simulink model "fs9_sim_sdr_v1"  (R2022b)
settings: Solver=ode4  StartTime=0.0  StopTime=dm.duration  FixedStep=dm.dt  RelTol=1e-3
PreLoadFcn:
  | addpath('./Common');
  | addpath('./design_tuning');
  | addpath('./sim_config');
  | addpath('./sim_analysis');
  | addpath('./fsw_init');
  | addpath('./mdls');
  | rads2rpm    = 60/(2*pi);  %rad/s to rpm
  | deg2rad     = pi/180;
  | set_mdl_variant;
InitFcn:
  | %b5g_init_param_sdr_v1;
model workspace (MAT data in the model file):
  RWModelType = 0
undefined symbols (not defined in the file or in its folder): dm, Eclipse, fsw, MagSc, mdl, PVeci, Qi2b, RateSc, SunSc
libraries: simulink x3, vrlib x2, aerolibtransform2 x1
(part 1 of 2)
Description:
  | This is a simplified model for B5G AOCS design and verification.
settings Model: SimulationMode=accelerator  PacingRate=501  ParameterArgumentNames=RWModelType  Creator=Jack-AOCS  LastModifiedBy=toby
settings SolverCC: AlgebraicLoopSolver=TrustRegion  MinimalZcImpactIntegration=on
settings DataIOCC: SaveFormat=Array
settings OptimizationCC: AccelVerboseBuild=on
settings DebuggingCC: ReadBeforeWriteMsg=DisableAll  WriteAfterWriteMsg=DisableAll  WriteAfterReadMsg=DisableAll  MultiTaskDSMMsg=none  UnconnectedInputMsg=warning  UnconnectedOutputMsg=warning  UnconnectedLineMsg=warning  SFMachineParentedDataDiag=warning  ArithmeticOperatorsInVariantConditions=warning
settings ModelReferenceCC: UpdateModelReferenceTargets=IfOutOfDate  EnableRefExpFcnMdlSchedulingChecks=on
settings SFSimCC: SFSimEcho=off  SimUseLocalCustomCode=off  CustomCodeUndefinedFunction=UseInterfaceOnly
settings RTWCC: RTWUseLocalCustomCode=off  DLArmComputeVersion=19.05

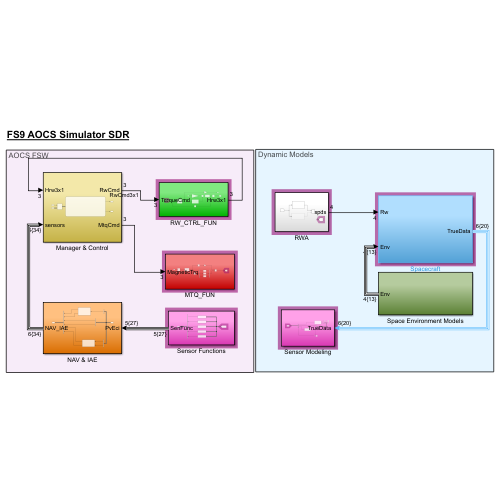
[thumbnail: Simulink's stored preview of the top-level diagram]
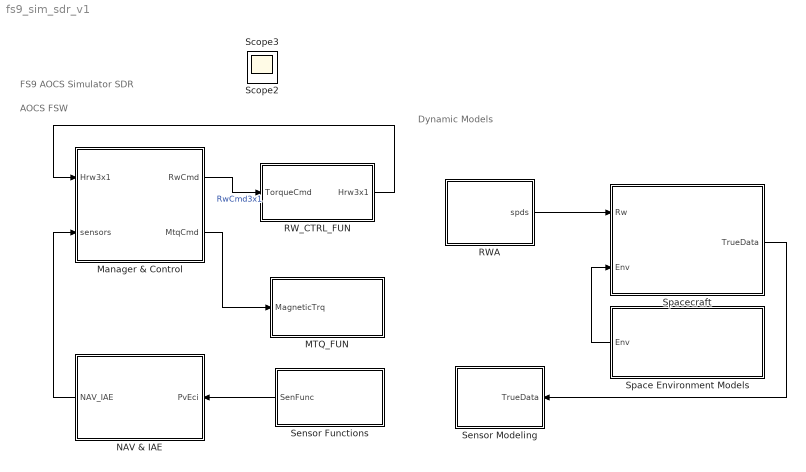
== system fs9_sim_sdr_v1 ==
  note: FS9 AOCS Simulator SDR
  note: AOCS FSW
  note: Dynamic Models
  MTQ_FUN : Subsystem
  Manager & Control : Subsystem
  NAV & IAE : Subsystem
  RWA : Subsystem
  RW_CTRL_FUN : Subsystem
  Sensor Functions : Subsystem
  Sensor Modeling : Subsystem
  Space Environment Models : Subsystem
  Spacecraft : Subsystem
  Scope2 : Scope
  Scope3 : Scope
  wires:
  RWA/1(spds) -> Spacecraft/1(Rw)
  Space Environment Models/1(Env) -> Spacecraft/2(Env)
  Spacecraft/1(TrueData) -> Sensor Modeling/1("TrueData ")
  RW_CTRL_FUN/1(Hrw3x1) -> Manager & Control/1(Hrw3x1)
  NAV & IAE/1(NAV_IAE) -> Manager & Control/2(sensors)
  Manager & Control/1(RwCmd) -> RW_CTRL_FUN/1(TorqueCmd)  "RwCmd3x1"
  Manager & Control/2(MtqCmd) -> MTQ_FUN/1(MagneticTrq)
  Sensor Functions/1(SenFunc) -> NAV & IAE/1(PvEci)

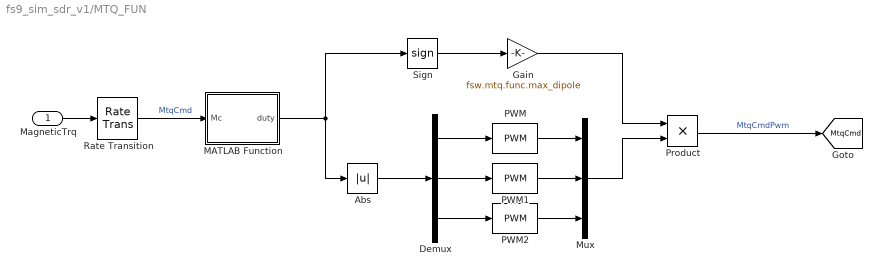
== system fs9_sim_sdr_v1/MTQ_FUN ==
  MagneticTrq : Inport
  Abs : Abs  SaturateOnIntegerOverflow=off
  Demux : Demux  Outputs=3
  Gain : Gain  Gain=fsw.mtq.func.max_dipole
  MATLAB Function : MATLAB Function  TreatAsAtomicUnit=on
  Mux : Mux  Inputs=3
  PWM : simulink/Discontinuities/PWM  DisableCoverage=on  Period=10  InitialDelay=0  DisallowZeroDutyCycle=off  RunAtFixedTimeIntervals=on  SampleTime=dm.dt
  PWM1 : simulink/Discontinuities/PWM  DisableCoverage=on  Period=10  InitialDelay=0  DisallowZeroDutyCycle=off  RunAtFixedTimeIntervals=on  SampleTime=dm.dt
  PWM2 : simulink/Discontinuities/PWM  DisableCoverage=on  Period=10  InitialDelay=0  DisallowZeroDutyCycle=off  RunAtFixedTimeIntervals=on  SampleTime=dm.dt
  Product : Product
  Rate Transition : RateTransition  OutPortSampleTime=fsw.mtq.cycle
  Sign : Signum
  tag scope: MtqCmd=global
  wires:
  Rate Transition/1 -> MATLAB Function/1(Mc)  "MtqCmd"
  Product/1 -> [MtqCmd]  "MtqCmdPwm"
  MagneticTrq/1 -> Rate Transition/1
  MATLAB Function/1(duty) -> Abs/1, Sign/1
  Abs/1 -> Demux/1
  Demux/1 -> PWM/1
  Demux/2 -> PWM1/1
  Demux/3 -> PWM2/1
  Sign/1 -> Gain/1
  PWM/1 -> Mux/1
  PWM1/1 -> Mux/2
  PWM2/1 -> Mux/3
  Gain/1 -> Product/1
  Mux/1 -> Product/2

== system fs9_sim_sdr_v1/Manager & Control ==
  Hrw3x1 : Inport
  sensors : Inport  Port=2
  AOCS_FSW : Stateflow chart  TreatAsAtomicUnit=on  SystemSampleTime=fsw.dt
  SENSOR_BUS : Subsystem
  RwCmd : Outport
  MtqCmd : Outport  Port=2
  wires:
  AOCS_FSW/1(RW_FUN) -> RwCmd/1  "RwTrq3"
  AOCS_FSW/2(MTQ_FUN) -> MtqCmd/1  "mtq_cmd"
  Hrw3x1/1 -> SENSOR_BUS/1(In1)
  sensors/1 -> SENSOR_BUS/2(In2)
  SENSOR_BUS/1(Out1) -> AOCS_FSW/1(SENSOR_IN)

== system fs9_sim_sdr_v1/NAV & IAE ==
  PvEci : Inport
  Bus Creator : BusCreator  Inputs=6
  Bus Selector1 : BusSelector  OutputSignals=GPS_FUNC
  Bus Selector2 : BusSelector  OutputSignals=STR_FUNC,GYRO_FUNC
  Bus Selector3 : BusSelector  OutputSignals=MAG_FUNC,SS_FUNC
  Inertial Attitude Estimation : MATLAB Function  TreatAsAtomicUnit=on  SystemSampleTime=fsw.dt
  NAVIGATION : MATLAB Function  TreatAsAtomicUnit=on  SystemSampleTime=fsw.dt
  NAV_IAE : Outport
  wires:
  Bus Selector1/1 -> NAVIGATION/1(pvt_eci)  "<GPS_FUNC>"
  PvEci/1 -> Bus Selector1/1, Bus Selector2/1, Bus Selector3/1
  NAVIGATION/1(nav_out) -> Bus Creator/1
  Bus Creator/1 -> NAV_IAE/1
  Bus Selector2/1 -> Inertial Attitude Estimation/1(Qi2b_true)  "<STR_FUNC>"
  Bus Selector2/2 -> Inertial Attitude Estimation/2(RateSc_true)  "<GYRO_FUNC>"
  Inertial Attitude Estimation/1(Q2ib) -> Bus Creator/5  "qi2b_est"
  Inertial Attitude Estimation/2(RateSc) -> Bus Creator/6  "rate_est"
  NAVIGATION/2(pvt_eci_nav) -> Bus Creator/2  "pvt_eci_nav"
  Bus Selector3/1 -> Bus Creator/3  "<MAG_FUNC>"
  Bus Selector3/2 -> Bus Creator/4  "<SS_FUNC>"

== system fs9_sim_sdr_v1/RWA ==
  Manual Switch : ManualSwitch
  "RWA " : Subsystem
  RWA with TorqueBox : Subsystem  Commented=on
  spds : Outport
  tag scope: RwSpds=global
  wires:
  [RwCmd] -> RWA with TorqueBox/1(In1), "RWA "/1(In1)
  RWA with TorqueBox/1(RW spd) -> Manual Switch/2
  "RWA "/1(RW spd) -> Manual Switch/1
  Manual Switch/1 -> [RwSpds], spds/1

== system fs9_sim_sdr_v1/RW_CTRL_FUN ==
  TorqueCmd : Inport
  Angular momentum Estimate : MATLAB Function  TreatAsAtomicUnit=on
  ComputeSaturate : MATLAB Function  TreatAsAtomicUnit=on
  D : Gain  Gain=fsw.rw.func.D  Multiplication=Matrix(K*u) (u vector)
  G : Gain  Gain=fsw.rw.func.G  Multiplication=Matrix(K*u) (u vector)
  RW Kernel Control : Subsystem
  Rate Transition : RateTransition  OutPortSampleTime=fsw.dt
  Sum2 : Sum  Inputs=|++
  Unit Delay : UnitDelay  SampleTime=-1  HasFrameUpgradeWarning=on
  Hrw3x1 : Outport
  tag scope: RwCmd=global
  wires:
  TorqueCmd/1 -> G/1
  [RwSpds] -> Angular momentum Estimate/1(w_rpm)  "RwSpd"
  G/1 -> Sum2/1  "C_A"
  Sum2/1 -> ComputeSaturate/1(T)
  Angular momentum Estimate/1(h) -> D/1, RW Kernel Control/1(h_est)  "h_est"
  Unit Delay/1 -> Angular momentum Estimate/2(tc)
  RW Kernel Control/1(C_N) -> Sum2/2
  ComputeSaturate/1(Tc) -> Rate Transition/1, Unit Delay/1
  Rate Transition/1 -> [RwCmd]  "RwTrq4"
  D/1 -> Hrw3x1/1  "Hrw"

== system fs9_sim_sdr_v1/Sensor Functions ==
  Bus Creator1 : BusCreator  Inputs=5
  GPS FUNCTION : Subsystem
  GYRO FUNCTION : Subsystem
  MAG FUNCTION : Subsystem
  SS FUNCTION : Subsystem
  STR FUNCTION : Subsystem
  SenFunc : Outport
  wires:
  [Sensors] -> SS FUNCTION/1("Hw "), MAG FUNCTION/1(Hw), GPS FUNCTION/1("Hw "), STR FUNCTION/1("Hw "), GYRO FUNCTION/1("Hw ")
  MAG FUNCTION/1(MAG_FUNC) -> Bus Creator1/1  "MAG_FUNC"
  Bus Creator1/1 -> SenFunc/1
  SS FUNCTION/1(SS_FUNC) -> Bus Creator1/2  "SS_FUNC"
  GYRO FUNCTION/1(GYRO_FUNC) -> Bus Creator1/3  "GYRO_FUNC"
  STR FUNCTION/1(STR_FUNC) -> Bus Creator1/4  "STR_FUNC"
  GPS FUNCTION/1(GPS_FUNC) -> Bus Creator1/5  "GPS_FUNC"

== system fs9_sim_sdr_v1/Sensor Modeling ==
  "TrueData " : Inport
  Bus Creator : BusCreator  Inputs=5
  Bus Selector : BusSelector  OutputSignals=SunSc,Eclipse
  Bus Selector1 : BusSelector  OutputSignals=RateSc,Qi2b,MagSc,PVeci
  MATLAB Function : MATLAB Function  TreatAsAtomicUnit=on
  Mux : Mux  Inputs=2
  Random Number : RandomNumber  Mean=[0 0]  Variance=[dm.ss_mdl.noise dm.ss_mdl.noise]'.^2  Seed=[0 1]  SampleTime=dm.dt
  ZARM FGM-A-75 : MATLAB Function  TreatAsAtomicUnit=on
  noise_enable : Gain  Gain=dm.ss_mdl.noise_enable
  tag scope: Sensors=global
  wires:
  "TrueData "/1 -> Bus Selector1/1, Bus Selector/1
  Bus Selector/1 -> MATLAB Function/2(SunSc)  "<SunSc>"
  Bus Selector/2 -> MATLAB Function/3(EclipFlag)  "<Eclipse>"
  MATLAB Function/1(SS_TM) -> Bus Creator/1
  Bus Selector1/1 -> Bus Creator/2  "<RateSc>"
  Bus Selector1/2 -> Bus Creator/3  "<Qi2b>"
  Bus Creator/1 -> [Sensors]
  [JD] -> Mux/2
  Bus Selector1/4 -> Mux/1  "<PVeci>"
  Mux/1 -> Bus Creator/5  "PVTeci"
  Random Number/1 -> noise_enable/1
  noise_enable/1 -> MATLAB Function/1(noise_ang)
  Bus Selector1/3 -> ZARM FGM-A-75/1(MagScTrue)  "<MagSc>"
  ZARM FGM-A-75/1(MagScNoise) -> Bus Creator/4

== system fs9_sim_sdr_v1/Space Environment Models ==
  Bus Creator : BusCreator  Inputs=4
  ECI2ECF : MATLAB Function  TreatAsAtomicUnit=on
  Eclipse Condition : MATLAB Function  TreatAsAtomicUnit=on
  MagneticField : Subsystem
  Mux : Mux  Inputs=2
  "Orbit Propagator " : Subsystem
  Product : Product  Multiplication=Matrix(*)
  Sun Model : MATLAB Function  TreatAsAtomicUnit=on
  Timer : Subsystem
  Env : Outport  VectorParamsAs1DForOutWhenUnconnected=off
  wires:
  ECI2ECF/1(Rf2i) -> Product/1
  Product/1 -> Bus Creator/1  "Beci"
  "Orbit Propagator "/1(Peci) -> ECI2ECF/2(Peci), Mux/1
  "Orbit Propagator "/2(Veci) -> Mux/2
  Timer/1(JD) -> Sun Model/1(jD), ECI2ECF/1(jdut1)
  Mux/1 -> Eclipse Condition/2(PvEci), Bus Creator/4  "PVeci"
  Bus Creator/1 -> Env/1
  Sun Model/1(SunEci) -> Bus Creator/2, Eclipse Condition/1(SunEci)  "SunVeci"
  Eclipse Condition/1(EclipFlag) -> Bus Creator/3  "Eclipse"
  ECI2ECF/2(Pecf) -> MagneticField/1(In1)
  MagneticField/1(Out1) -> Product/2

== system fs9_sim_sdr_v1/Spacecraft ==
  Rw : Inport
  Env : Inport  Port=2
  EPS : Subsystem
  Spacecraft Dynamics : Subsystem
  TrueData : Outport  VectorParamsAs1DForOutWhenUnconnected=off
  wires:
  [MtqCmd] -> Spacecraft Dynamics/1(Mtq)
  Rw/1 -> Spacecraft Dynamics/2(Rw)  "RwSpd"
  Env/1 -> Spacecraft Dynamics/3(In3)
  Spacecraft Dynamics/1(Out1) -> EPS/1(In1), TrueData/1

== system fs9_sim_sdr_v1/Manager & Control/AOCS_FSW/AOCS_MGR.ASH_MGR.magnetic_control ==
  MAG_FUNC : Inport  OutDataTypeStr=double  PortDimensions=9
  f : TriggerPort  TriggerType=function-call  VariantControl=(inherit)
      settings: CopyFcn=Stateflow.SLINSF.SimulinkMan.removeBlockPreDeleteFcn  PreDeleteFcn=Stateflow.SLINSF.SimulinkMan.unsafePredeleteFcn
  Bdot Control : MATLAB Function  TreatAsAtomicUnit=on
  mtq_cmd : Outport
  wires:
  MAG_FUNC/1 -> Bdot Control/1(MAG_FUNC)  "mag_func"
  Bdot Control/1(Mc) -> mtq_cmd/1  "M"

== system fs9_sim_sdr_v1/Manager & Control/AOCS_FSW/AOCS_MGR.ASH_MGR.rw_momentum_control ==
  HrwEst : Inport  OutDataTypeStr=double  PortDimensions=3
  f : TriggerPort  TriggerType=function-call  VariantControl=(inherit)
      settings: CopyFcn=Stateflow.SLINSF.SimulinkMan.removeBlockPreDeleteFcn  PreDeleteFcn=Stateflow.SLINSF.SimulinkMan.unsafePredeleteFcn
  Kernel momentum gain(H_used) : Gain  Gain=fsw.ash_ctrl.total_ang_mom_gain
  Sum : Sum  Inputs=|+-
  zero_spd_cmd(H_used) : Constant  Value=fsw.ash_ctrl.angular_mom_dir * fsw.ash_ctrl.cur_total_ang_mom_ref
  rw_cmd : Outport
  wires:
  zero_spd_cmd(H_used)/1 -> Sum/1
  Kernel momentum gain(H_used)/1 -> rw_cmd/1  "bias_torque_cmd"
  HrwEst/1 -> Sum/2  "Total angular moementum"
  Sum/1 -> Kernel momentum gain(H_used)/1

== system fs9_sim_sdr_v1/Manager & Control/AOCS_FSW/AOCS_MGR.ASH_MGR.stop_sim ==
  f : TriggerPort  TriggerType=function-call  VariantControl=(inherit)
      settings: CopyFcn=Stateflow.SLINSF.SimulinkMan.removeBlockPreDeleteFcn  PreDeleteFcn=Stateflow.SLINSF.SimulinkMan.unsafePredeleteFcn
  Constant : Constant
  Stop Simulation : Stop
  wires:
  Constant/1 -> Stop Simulation/1

== system fs9_sim_sdr_v1/Manager & Control/AOCS_FSW/AOCS_MGR.ASH_MGR.sunsensor_control ==
  ss_tm : Inport  OutDataTypeStr=double  PortDimensions=4
  iru_tm : Inport  Port=2  OutDataTypeStr=double  PortDimensions=3
  f : TriggerPort  TriggerType=function-call  VariantControl=(inherit)
      settings: CopyFcn=Stateflow.SLINSF.SimulinkMan.removeBlockPreDeleteFcn  PreDeleteFcn=Stateflow.SLINSF.SimulinkMan.unsafePredeleteFcn
  Sun Capture Controller : Subsystem
  SunAngErr : MATLAB Function  TreatAsAtomicUnit=on
  rw_cmd : Outport
  wires:
  Sun Capture Controller/1(RW_FUN) -> rw_cmd/1
  SunAngErr/1(deltaAngle_c2b) -> Sun Capture Controller/1(deltaAngle_c2b)  "DltAngeC2B"
  iru_tm/1 -> Sun Capture Controller/2(IRU_FUN)
  ss_tm/1 -> SunAngErr/1(snr_fun)

== system fs9_sim_sdr_v1/Manager & Control/SENSOR_BUS ==
  In1 : Inport
  In2 : Inport  Port=2
  Bus Creator : BusCreator  Inputs=7  OutDataTypeStr=Bus: SENSORS
  Bus Selector : BusSelector  OutputSignals=MAG_FUNC,SS_FUNC,rate_est,qi2b_est,pvt_eci_nav,nav_out
  Rate Transition : RateTransition  OutPortSampleTime=fsw.dt
  Out1 : Outport
  wires:
  In2/1 -> Bus Selector/1
  Bus Selector/3 -> Bus Creator/4  "<rate_est>"
  Bus Selector/2 -> Bus Creator/3  "<SS_FUNC>"
  In1/1 -> Bus Creator/1
  Bus Selector/5 -> Bus Creator/6  "<pvt_eci_nav>"
  Bus Selector/4 -> Bus Creator/5  "<qi2b_est>"
  Bus Selector/1 -> Bus Creator/2  "<MAG_FUNC>"
  Bus Selector/6 -> Bus Creator/7  "<nav_out>"
  Bus Creator/1 -> Rate Transition/1
  Rate Transition/1 -> Out1/1

== system fs9_sim_sdr_v1/RWA/RWA  ==
  In1 : Inport
  Demux : Demux
  Mux : Mux
  RW1 : Subsystem
  RW2 : Subsystem
  RW3 : Subsystem
  RW4 : Subsystem
  RW spd : Outport
  wires:
  RW3/1(Out1) -> Mux/3
  RW4/1(Out1) -> Mux/4
  Demux/4 -> RW4/1(torque_cmd)
  Demux/1 -> RW1/1(torque_cmd)
  Demux/2 -> RW2/1(torque_cmd)
  Demux/3 -> RW3/1(torque_cmd)
  RW2/1(Out1) -> Mux/2
  RW1/1(Out1) -> Mux/1
  Mux/1 -> RW spd/1  "RW spd"
  In1/1 -> Demux/1

== system fs9_sim_sdr_v1/RWA/RWA with TorqueBox ==
  In1 : Inport
  Demux : Demux
  Mux : Mux
  RW1 : Subsystem
  RW2 : Subsystem
  RW3 : Subsystem
  RW4 : Subsystem
  RW spd : Outport
  wires:
  RW1/1(Out1) -> Mux/1
  Demux/1 -> RW1/1(torque_cmd)
  Demux/3 -> RW3/1(torque_cmd)
  RW2/1(Out1) -> Mux/2
  Demux/4 -> RW4/1(torque_cmd)
  RW3/1(Out1) -> Mux/3
  Mux/1 -> RW spd/1  "RW spd"
  Demux/2 -> RW2/1(torque_cmd)
  RW4/1(Out1) -> Mux/4
  In1/1 -> Demux/1

== system fs9_sim_sdr_v1/RW_CTRL_FUN/RW Kernel Control ==
  h_est : Inport
  Kernel angular momentum(h_used) : Constant  Value=fsw.rw.func.KERNEL_ANG_MOM_REF
  Kernel direction : Gain  Gain=fsw.rw.func.K_KERNEL_DIRECTION
  Kernel momentum gain(h_used) : Gain  Gain=fsw.rw.func.KERNEL_ANG_MOM_GAIN
  Sum3 : Sum  Inputs=|+-
  kernal angular moementum : Gain  Gain=fsw.rw.func.E  Multiplication=Matrix(K*u) (u vector)
  C_N : Outport
  wires:
  Kernel angular momentum(h_used)/1 -> Kernel direction/1
  Kernel direction/1 -> Sum3/1  "hc"
  kernal angular moementum/1 -> Sum3/2
  Kernel momentum gain(h_used)/1 -> C_N/1  "C_N"
  Sum3/1 -> Kernel momentum gain(h_used)/1
  h_est/1 -> kernal angular moementum/1

== system fs9_sim_sdr_v1/Sensor Functions/GPS FUNCTION ==
  "Hw " : Inport
  Bus Selector : BusSelector  OutputSignals=PVTeci
  GPS_FUNC : Outport
  wires:
  Bus Selector/1 -> GPS_FUNC/1  "<PVTeci>"
  "Hw "/1 -> Bus Selector/1

== system fs9_sim_sdr_v1/Sensor Functions/GYRO FUNCTION ==
  "Hw " : Inport
  Bus Selector : BusSelector  OutputSignals=RateSc
  GYRO_FUNC : Outport
  wires:
  Bus Selector/1 -> GYRO_FUNC/1  "<RateSc>"
  "Hw "/1 -> Bus Selector/1

== system fs9_sim_sdr_v1/Sensor Functions/MAG FUNCTION ==
  Hw : Inport
  Bus Selector : BusSelector  OutputSignals=MagScNoise
  Discrete SOF : DiscreteTransferFcn  Numerator=fsw.ash.sof.num  Denominator=fsw.ash.sof.den
  Mux : Mux  Inputs=3
  Rate Transition : RateTransition  OutPortSampleTime=fsw.bdot_period
  Reshape : Reshape
  Reshape1 : Reshape
  bdotsdot : MATLAB Function  TreatAsAtomicUnit=on
  MAG_FUNC : Outport
  wires:
  Bus Selector/1 -> Rate Transition/1  "<MagScNoise>"
  bdotsdot/1(bdot) -> Discrete SOF/1
  Discrete SOF/1 -> Mux/1  "udot"
  Mux/1 -> MAG_FUNC/1  "MAG_FUNC"
  bdotsdot/2(sdot) -> Reshape/1  "sdot"
  Hw/1 -> Bus Selector/1
  Rate Transition/1 -> Reshape1/1, bdotsdot/1(B)
  Reshape/1 -> Mux/2
  Reshape1/1 -> Mux/3  "MagMeasSc"

== system fs9_sim_sdr_v1/Sensor Functions/SS FUNCTION ==
  "Hw " : Inport
  Bus Selector : BusSelector  OutputSignals=SS_TM
  SS_FUNC : Outport
  wires:
  "Hw "/1 -> Bus Selector/1
  Bus Selector/1 -> SS_FUNC/1  "<SS_TM>"

== system fs9_sim_sdr_v1/Sensor Functions/STR FUNCTION ==
  "Hw " : Inport
  Bus Selector : BusSelector  OutputSignals=Qi2b
  STR_FUNC : Outport
  wires:
  "Hw "/1 -> Bus Selector/1
  Bus Selector/1 -> STR_FUNC/1  "<Qi2b>"

== system fs9_sim_sdr_v1/Space Environment Models/MagneticField ==
  In1 : Inport
  Variant Subsystem : Subsystem  Variant=on
  Out1 : Outport
  wires:
  In1/1 -> Variant Subsystem/1(Pecf)
  Variant Subsystem/1(BnT) -> Out1/1

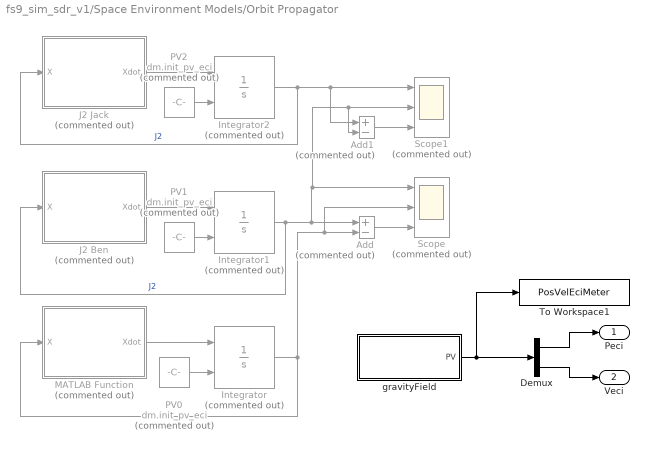
== system fs9_sim_sdr_v1/Space Environment Models/Orbit Propagator  ==
  Add : Sum  Commented=on  Inputs=+-
  Add1 : Sum  Commented=on  Inputs=+-
  Demux : Demux  Outputs=2
  Integrator : Integrator  Commented=on  InitialConditionSource=external
  Integrator1 : Integrator  Commented=on  InitialConditionSource=external
  Integrator2 : Integrator  Commented=on  InitialConditionSource=external
  J2 Ben : MATLAB Function  Commented=on  TreatAsAtomicUnit=on
  J2 Jack : MATLAB Function  Commented=on  TreatAsAtomicUnit=on
  MATLAB Function : MATLAB Function  Commented=on  TreatAsAtomicUnit=on
  PV0 : Constant  Commented=on  Value=dm.init_pv_eci
  PV1 : Constant  Commented=on  Value=dm.init_pv_eci
  PV2 : Constant  Commented=on  Value=dm.init_pv_eci
  Scope : Scope  Commented=on  NumInputPorts=3
  Scope1 : Scope  Commented=on  NumInputPorts=3
  To Workspace1 : ToWorkspace  VariableName=PosVelEciMeter  SaveFormat=Timeseries  SampleTime=-1
  gravityField : Subsystem  Variant=on
  Peci : Outport  VectorParamsAs1DForOutWhenUnconnected=off
  Veci : Outport  Port=2  VectorParamsAs1DForOutWhenUnconnected=off
  wires:
  Demux/2 -> Veci/1
  MATLAB Function/1(Xdot) -> Integrator/1
  Integrator/1 -> Add/2, Scope/2, MATLAB Function/1(X)
  Demux/1 -> Peci/1
  PV0/1 -> Integrator/2
  PV1/1 -> Integrator1/2
  J2 Ben/1(Xdot) -> Integrator1/1
  Integrator1/1 -> J2 Ben/1(X), Add/1, Add1/2, Scope1/2, Scope/1  "J2"
  Add/1 -> Scope/3
  PV2/1 -> Integrator2/2
  J2 Jack/1(Xdot) -> Integrator2/1
  Integrator2/1 -> J2 Jack/1(X), Add1/1, Scope1/1  "J2"
  Add1/1 -> Scope1/3
  gravityField/1(PV) -> To Workspace1/1, Demux/1

== system fs9_sim_sdr_v1/Space Environment Models/Timer ==
  Clock : Clock
  Constant : Constant  Value=dm.jd0
  Gain : Gain  Gain=1/86400
  Sum : Sum  Inputs=|++
  JD : Outport  VectorParamsAs1DForOutWhenUnconnected=off
  tag scope: JD=global
  wires:
  Clock/1 -> Gain/1
  Gain/1 -> Sum/2
  Constant/1 -> Sum/1
  Sum/1 -> [JD], JD/1

== system fs9_sim_sdr_v1/Spacecraft/EPS ==
  In1 : Inport
  Bus Selector : BusSelector  OutputSignals=Eclipse,SunSc
  DOD Calculation : MATLAB Function  TreatAsAtomicUnit=on
  Terminator{,1..3} (4 alike) : Terminator
  wires:
  In1/1 -> Bus Selector/1
  Bus Selector/1 -> DOD Calculation/1(eclipse_flag)  "<Eclipse>"
  Bus Selector/2 -> DOD Calculation/2(sun_sc)  "<SunSc>"
  DOD Calculation/1(dod) -> Terminator/1  "dod"
  DOD Calculation/2(dod_max) -> Terminator1/1  "dod_max"
  DOD Calculation/3(sa_ang) -> Terminator2/1  "sa_ang"
  DOD Calculation/4(batt_io_energy) -> Terminator3/1  "batt_io_energy"

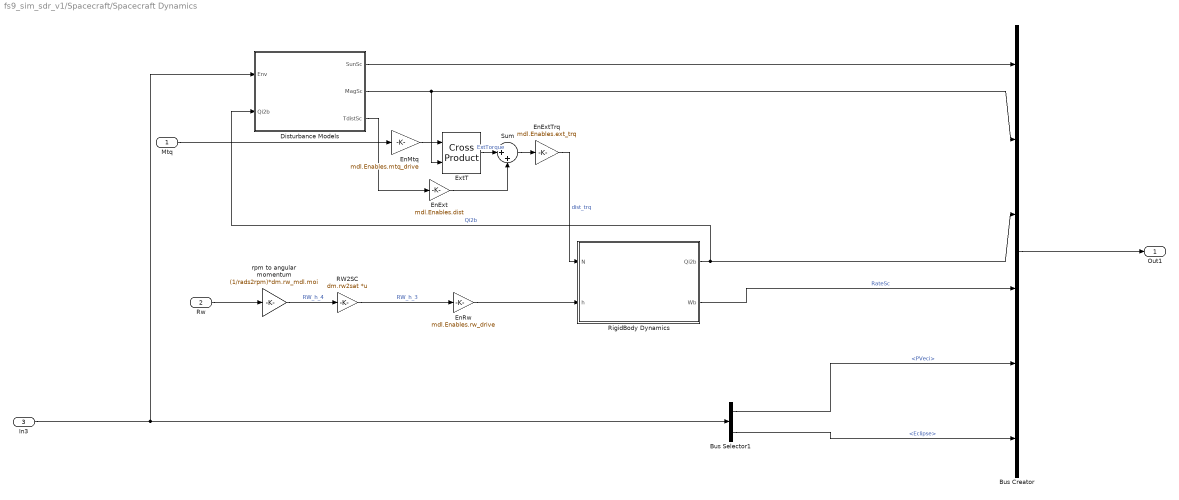
== system fs9_sim_sdr_v1/Spacecraft/Spacecraft Dynamics ==
  Mtq : Inport
  Rw : Inport  Port=2
  In3 : Inport  Port=3
  Bus Creator : BusCreator  Inputs=SunSc,MagSc,Qi2b,RateSc,PVeci,Eclipse
  Bus Selector1 : BusSelector  OutputSignals=PVeci,Eclipse
  Disturbance Models : Subsystem
  EnExt : Gain  Gain=mdl.Enables.dist
  EnExtTrq : Gain  Gain=mdl.Enables.ext_trq
  EnMtq : Gain  Gain=mdl.Enables.mtq_drive
  EnRw : Gain  Gain=mdl.Enables.rw_drive
  ExtT : vrlib/Utilities/Cross Product
  RW2SC : Gain  Gain=dm.rw2sat  Multiplication=Matrix(K*u)
  RigidBody Dynamics : Subsystem
  Sum : Sum  Inputs=|++
  rpm to angular momentum : Gain  Gain=(1/rads2rpm)*dm.rw_mdl.moi
  Out1 : Outport
  wires:
  RW2SC/1 -> EnRw/1  "RW_h_3"
  RigidBody Dynamics/1(Qi2b) -> Disturbance Models/2(Qi2b), Bus Creator/3  "Qi2b"
  ExtT/1 -> Sum/1  "ExtTorque"
  Sum/1 -> EnExtTrq/1
  Bus Selector1/1 -> Bus Creator/5  "<PVeci>"
  Rw/1 -> rpm to angular momentum/1
  EnExt/1 -> Sum/2
  Mtq/1 -> EnMtq/1
  In3/1 -> Disturbance Models/1(Env), Bus Selector1/1
  EnRw/1 -> RigidBody Dynamics/2(h)
  RigidBody Dynamics/2(Wb) -> Bus Creator/4  "RateSc"
  Bus Selector1/2 -> Bus Creator/6  "<Eclipse>"
  Disturbance Models/3(TdistSc) -> EnExt/1
  Disturbance Models/2(MagSc) -> Bus Creator/2, ExtT/2
  rpm to angular momentum/1 -> RW2SC/1  "RW_h_4"
  Disturbance Models/1(SunSc) -> Bus Creator/1
  EnMtq/1 -> ExtT/1
  EnExtTrq/1 -> RigidBody Dynamics/1(N)  "dist_trq"
  Bus Creator/1 -> Out1/1

== system fs9_sim_sdr_v1/Manager & Control/AOCS_FSW/AOCS_MGR.ASH_MGR.sunsensor_control/Sun Capture Controller ==
  note: SunCapture Controller Design
  deltaAngle_c2b : Inport
  IRU_FUN : Inport  Port=2
  KD : Gain  Gain=fsw.RLPD.kd
  KP : Gain  Gain=fsw.RLPD.kp
  Saturation : Saturate  UpperLimit=0.02  LowerLimit=-0.02
  Sum : Sum  Inputs=|++
  RW_FUN : Outport  VectorParamsAs1DForOutWhenUnconnected=off
  wires:
  Saturation/1 -> Sum/1  "CmdKp"
  KP/1 -> Saturation/1
  KD/1 -> RW_FUN/1  "tapd_rw_cmd"
  Sum/1 -> KD/1
  deltaAngle_c2b/1 -> KP/1
  IRU_FUN/1 -> Sum/2

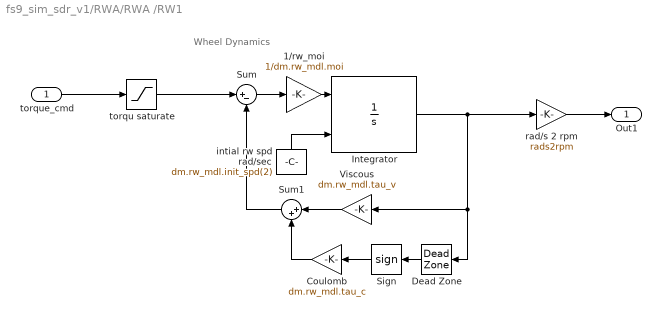
== system fs9_sim_sdr_v1/RWA/RWA /RW1 ==
  note: Wheel Dynamics
  torque_cmd : Inport
  1/rw_moi : Gain  Gain=1/dm.rw_mdl.moi
  Coulomb : Gain  Gain=dm.rw_mdl.tau_c
  Dead Zone : DeadZone  LowerValue=-dm.rw_mdl.dead_zone  UpperValue=dm.rw_mdl.dead_zone  SaturateOnIntegerOverflow=off
  Integrator : Integrator  InitialConditionSource=external
  Sign : Signum
  Sum : Sum  Inputs=|+-
  Sum1 : Sum  Inputs=|++
  Viscous : Gain  Gain=dm.rw_mdl.tau_v
  intial rw spd rad/sec : Constant  Value=dm.rw_mdl.init_spd(2)
  rad/s 2 rpm : Gain  Gain=rads2rpm
  torqu saturate : Saturate  UpperLimit=dm.rw_mdl.maxTorque  LowerLimit=-dm.rw_mdl.maxTorque
  Out1 : Outport
  wires:
  rad/s 2 rpm/1 -> Out1/1
  Sum1/1 -> Sum/2
  torqu saturate/1 -> Sum/1
  1/rw_moi/1 -> Integrator/1
  Sign/1 -> Coulomb/1
  Coulomb/1 -> Sum1/2
  intial rw spd rad/sec/1 -> Integrator/2
  Sum/1 -> 1/rw_moi/1
  torque_cmd/1 -> torqu saturate/1
  Integrator/1 -> Dead Zone/1, Viscous/1, rad/s 2 rpm/1
  Viscous/1 -> Sum1/1
  Dead Zone/1 -> Sign/1

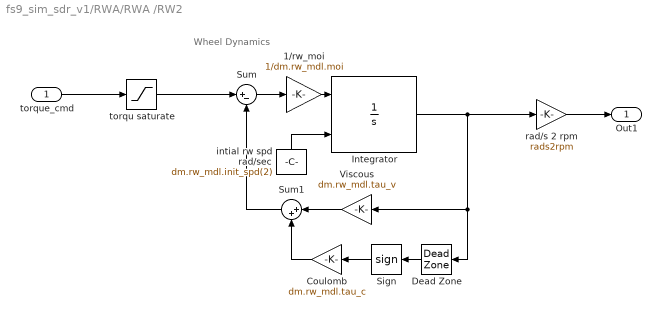
== system fs9_sim_sdr_v1/RWA/RWA /RW2 ==
  note: Wheel Dynamics
  torque_cmd : Inport
  1/rw_moi : Gain  Gain=1/dm.rw_mdl.moi
  Coulomb : Gain  Gain=dm.rw_mdl.tau_c
  Dead Zone : DeadZone  LowerValue=-dm.rw_mdl.dead_zone  UpperValue=dm.rw_mdl.dead_zone  SaturateOnIntegerOverflow=off
  Integrator : Integrator  InitialConditionSource=external
  Sign : Signum
  Sum : Sum  Inputs=|+-
  Sum1 : Sum  Inputs=|++
  Viscous : Gain  Gain=dm.rw_mdl.tau_v
  intial rw spd rad/sec : Constant  Value=dm.rw_mdl.init_spd(2)
  rad/s 2 rpm : Gain  Gain=rads2rpm
  torqu saturate : Saturate  UpperLimit=dm.rw_mdl.maxTorque  LowerLimit=-dm.rw_mdl.maxTorque
  Out1 : Outport
  wires:
  Dead Zone/1 -> Sign/1
  Viscous/1 -> Sum1/1
  Integrator/1 -> rad/s 2 rpm/1, Viscous/1, Dead Zone/1
  torque_cmd/1 -> torqu saturate/1
  Sum/1 -> 1/rw_moi/1
  intial rw spd rad/sec/1 -> Integrator/2
  Coulomb/1 -> Sum1/2
  Sign/1 -> Coulomb/1
  1/rw_moi/1 -> Integrator/1
  torqu saturate/1 -> Sum/1
  Sum1/1 -> Sum/2
  rad/s 2 rpm/1 -> Out1/1

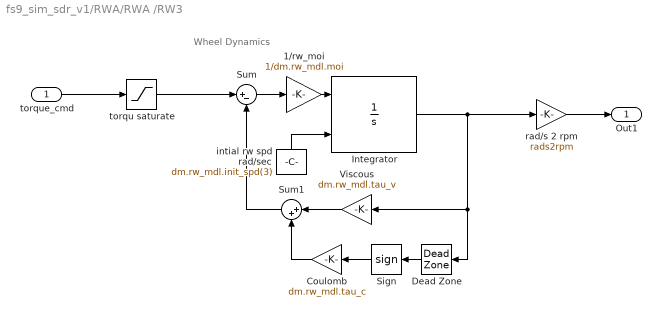
== system fs9_sim_sdr_v1/RWA/RWA /RW3 ==
  note: Wheel Dynamics
  torque_cmd : Inport
  1/rw_moi : Gain  Gain=1/dm.rw_mdl.moi
  Coulomb : Gain  Gain=dm.rw_mdl.tau_c
  Dead Zone : DeadZone  LowerValue=-dm.rw_mdl.dead_zone  UpperValue=dm.rw_mdl.dead_zone  SaturateOnIntegerOverflow=off
  Integrator : Integrator  InitialConditionSource=external
  Sign : Signum
  Sum : Sum  Inputs=|+-
  Sum1 : Sum  Inputs=|++
  Viscous : Gain  Gain=dm.rw_mdl.tau_v
  intial rw spd rad/sec : Constant  Value=dm.rw_mdl.init_spd(3)
  rad/s 2 rpm : Gain  Gain=rads2rpm
  torqu saturate : Saturate  UpperLimit=dm.rw_mdl.maxTorque  LowerLimit=-dm.rw_mdl.maxTorque
  Out1 : Outport
  wires:
  Dead Zone/1 -> Sign/1
  Viscous/1 -> Sum1/1
  Integrator/1 -> rad/s 2 rpm/1, Viscous/1, Dead Zone/1
  torque_cmd/1 -> torqu saturate/1
  Sum/1 -> 1/rw_moi/1
  intial rw spd rad/sec/1 -> Integrator/2
  Coulomb/1 -> Sum1/2
  Sign/1 -> Coulomb/1
  1/rw_moi/1 -> Integrator/1
  torqu saturate/1 -> Sum/1
  Sum1/1 -> Sum/2
  rad/s 2 rpm/1 -> Out1/1

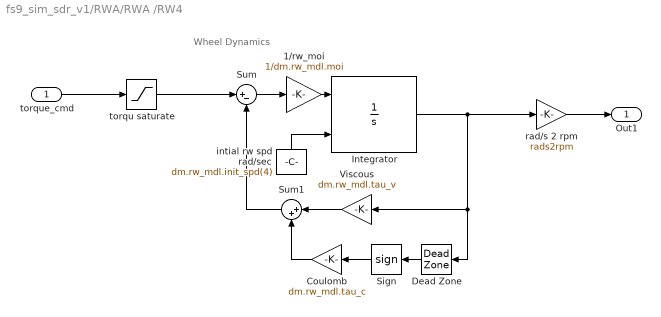
== system fs9_sim_sdr_v1/RWA/RWA /RW4 ==
  note: Wheel Dynamics
  torque_cmd : Inport
  1/rw_moi : Gain  Gain=1/dm.rw_mdl.moi
  Coulomb : Gain  Gain=dm.rw_mdl.tau_c
  Dead Zone : DeadZone  LowerValue=-dm.rw_mdl.dead_zone  UpperValue=dm.rw_mdl.dead_zone  SaturateOnIntegerOverflow=off
  Integrator : Integrator  InitialConditionSource=external
  Sign : Signum
  Sum : Sum  Inputs=|+-
  Sum1 : Sum  Inputs=|++
  Viscous : Gain  Gain=dm.rw_mdl.tau_v
  intial rw spd rad/sec : Constant  Value=dm.rw_mdl.init_spd(4)
  rad/s 2 rpm : Gain  Gain=rads2rpm
  torqu saturate : Saturate  UpperLimit=dm.rw_mdl.maxTorque  LowerLimit=-dm.rw_mdl.maxTorque
  Out1 : Outport
  wires:
  Dead Zone/1 -> Sign/1
  Viscous/1 -> Sum1/1
  Integrator/1 -> rad/s 2 rpm/1, Viscous/1, Dead Zone/1
  torque_cmd/1 -> torqu saturate/1
  Sum/1 -> 1/rw_moi/1
  intial rw spd rad/sec/1 -> Integrator/2
  Coulomb/1 -> Sum1/2
  Sign/1 -> Coulomb/1
  1/rw_moi/1 -> Integrator/1
  torqu saturate/1 -> Sum/1
  Sum1/1 -> Sum/2
  rad/s 2 rpm/1 -> Out1/1

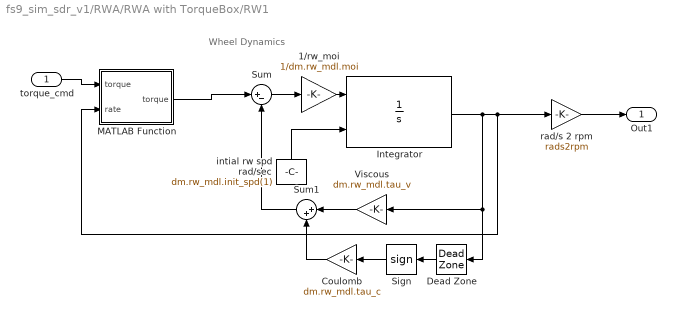
== system fs9_sim_sdr_v1/RWA/RWA with TorqueBox/RW1 ==
  note: Wheel Dynamics
  torque_cmd : Inport
  1/rw_moi : Gain  Gain=1/dm.rw_mdl.moi
  Coulomb : Gain  Gain=dm.rw_mdl.tau_c
  Dead Zone : DeadZone  LowerValue=-dm.rw_mdl.dead_zone  UpperValue=dm.rw_mdl.dead_zone  SaturateOnIntegerOverflow=off
  Integrator : Integrator  InitialConditionSource=external
  MATLAB Function : MATLAB Function  TreatAsAtomicUnit=on
  Sign : Signum
  Sum : Sum  Inputs=|+-
  Sum1 : Sum  Inputs=|++
  Viscous : Gain  Gain=dm.rw_mdl.tau_v
  intial rw spd rad/sec : Constant  Value=dm.rw_mdl.init_spd(1)
  rad/s 2 rpm : Gain  Gain=rads2rpm
  Out1 : Outport
  wires:
  Dead Zone/1 -> Sign/1
  Viscous/1 -> Sum1/1
  Integrator/1 -> MATLAB Function/2(rate), rad/s 2 rpm/1, Viscous/1, Dead Zone/1
  torque_cmd/1 -> MATLAB Function/1("torque ")
  Sum/1 -> 1/rw_moi/1
  intial rw spd rad/sec/1 -> Integrator/2
  Coulomb/1 -> Sum1/2
  Sign/1 -> Coulomb/1
  1/rw_moi/1 -> Integrator/1
  Sum1/1 -> Sum/2
  rad/s 2 rpm/1 -> Out1/1
  MATLAB Function/1(torque) -> Sum/1

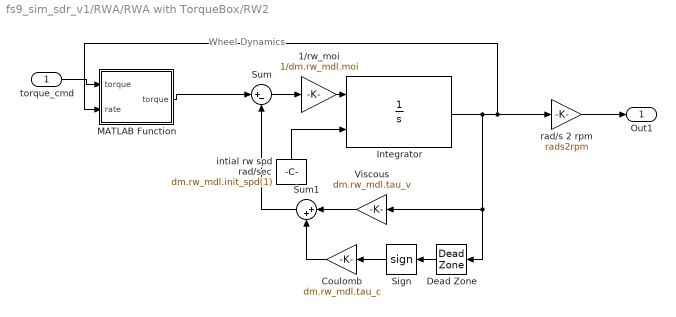
== system fs9_sim_sdr_v1/RWA/RWA with TorqueBox/RW2 ==
  note: Wheel Dynamics
  torque_cmd : Inport
  1/rw_moi : Gain  Gain=1/dm.rw_mdl.moi
  Coulomb : Gain  Gain=dm.rw_mdl.tau_c
  Dead Zone : DeadZone  LowerValue=-dm.rw_mdl.dead_zone  UpperValue=dm.rw_mdl.dead_zone  SaturateOnIntegerOverflow=off
  Integrator : Integrator  InitialConditionSource=external
  MATLAB Function : MATLAB Function  TreatAsAtomicUnit=on
  Sign : Signum
  Sum : Sum  Inputs=|+-
  Sum1 : Sum  Inputs=|++
  Viscous : Gain  Gain=dm.rw_mdl.tau_v
  intial rw spd rad/sec : Constant  Value=dm.rw_mdl.init_spd(1)
  rad/s 2 rpm : Gain  Gain=rads2rpm
  Out1 : Outport
  wires:
  Dead Zone/1 -> Sign/1
  Viscous/1 -> Sum1/1
  Integrator/1 -> MATLAB Function/2(rate), rad/s 2 rpm/1, Viscous/1, Dead Zone/1
  torque_cmd/1 -> MATLAB Function/1("torque ")
  Sum/1 -> 1/rw_moi/1
  intial rw spd rad/sec/1 -> Integrator/2
  Coulomb/1 -> Sum1/2
  Sign/1 -> Coulomb/1
  1/rw_moi/1 -> Integrator/1
  Sum1/1 -> Sum/2
  rad/s 2 rpm/1 -> Out1/1
  MATLAB Function/1(torque) -> Sum/1

== system fs9_sim_sdr_v1/RWA/RWA with TorqueBox/RW3 ==
  note: Wheel Dynamics
  torque_cmd : Inport
  1/rw_moi : Gain  Gain=1/dm.rw_mdl.moi
  Coulomb : Gain  Gain=dm.rw_mdl.tau_c
  Dead Zone : DeadZone  LowerValue=-dm.rw_mdl.dead_zone  UpperValue=dm.rw_mdl.dead_zone  SaturateOnIntegerOverflow=off
  Integrator : Integrator  InitialConditionSource=external
  MATLAB Function : MATLAB Function  TreatAsAtomicUnit=on
  Sign : Signum
  Sum : Sum  Inputs=|+-
  Sum1 : Sum  Inputs=|++
  Viscous : Gain  Gain=dm.rw_mdl.tau_v
  intial rw spd rad/sec : Constant  Value=dm.rw_mdl.init_spd(1)
  rad/s 2 rpm : Gain  Gain=rads2rpm
  Out1 : Outport
  wires:
  Dead Zone/1 -> Sign/1
  Viscous/1 -> Sum1/1
  Integrator/1 -> MATLAB Function/2(rate), rad/s 2 rpm/1, Viscous/1, Dead Zone/1
  torque_cmd/1 -> MATLAB Function/1("torque ")
  Sum/1 -> 1/rw_moi/1
  intial rw spd rad/sec/1 -> Integrator/2
  Coulomb/1 -> Sum1/2
  Sign/1 -> Coulomb/1
  1/rw_moi/1 -> Integrator/1
  Sum1/1 -> Sum/2
  rad/s 2 rpm/1 -> Out1/1
  MATLAB Function/1(torque) -> Sum/1

== system fs9_sim_sdr_v1/RWA/RWA with TorqueBox/RW4 ==
  note: Wheel Dynamics
  torque_cmd : Inport
  1/rw_moi : Gain  Gain=1/dm.rw_mdl.moi
  Coulomb : Gain  Gain=dm.rw_mdl.tau_c
  Dead Zone : DeadZone  LowerValue=-dm.rw_mdl.dead_zone  UpperValue=dm.rw_mdl.dead_zone  SaturateOnIntegerOverflow=off
  Integrator : Integrator  InitialConditionSource=external
  MATLAB Function : MATLAB Function  TreatAsAtomicUnit=on
  Sign : Signum
  Sum : Sum  Inputs=|+-
  Sum1 : Sum  Inputs=|++
  Viscous : Gain  Gain=dm.rw_mdl.tau_v
  intial rw spd rad/sec : Constant  Value=dm.rw_mdl.init_spd(1)
  rad/s 2 rpm : Gain  Gain=rads2rpm
  Out1 : Outport
  wires:
  Dead Zone/1 -> Sign/1
  Viscous/1 -> Sum1/1
  Integrator/1 -> MATLAB Function/2(rate), rad/s 2 rpm/1, Viscous/1, Dead Zone/1
  torque_cmd/1 -> MATLAB Function/1("torque ")
  Sum/1 -> 1/rw_moi/1
  intial rw spd rad/sec/1 -> Integrator/2
  Coulomb/1 -> Sum1/2
  Sign/1 -> Coulomb/1
  1/rw_moi/1 -> Integrator/1
  Sum1/1 -> Sum/2
  rad/s 2 rpm/1 -> Out1/1
  MATLAB Function/1(torque) -> Sum/1

== system fs9_sim_sdr_v1/Space Environment Models/MagneticField/Variant Subsystem ==
  note: 1) Add Subsystem or Model blocks as valid variant choices.
      | 2) You cannot connect blocks at this level. At simulation, connectivity is automatically
      | determined, based on the active variant and port name matching.
  Pecf : Inport
  IGRF2020 : Subsystem  VariantControl=M_IGRF
  MagneticDipoleModel : MATLAB Function  TreatAsAtomicUnit=on  VariantControl=M_DIPOLE
  BnT : Outport

== system fs9_sim_sdr_v1/Space Environment Models/Orbit Propagator /gravityField ==
  note: 1) Add Subsystem or Model blocks as valid variant choices.
      | 2) You cannot connect blocks at this level. At simulation, connectivity is automatically
      | determined, based on the active variant and port name matching.
  J2 : Subsystem  VariantControl=G_J2
  TwoBodyRHS : Subsystem  VariantControl=G_TwoBody
  PV : Outport

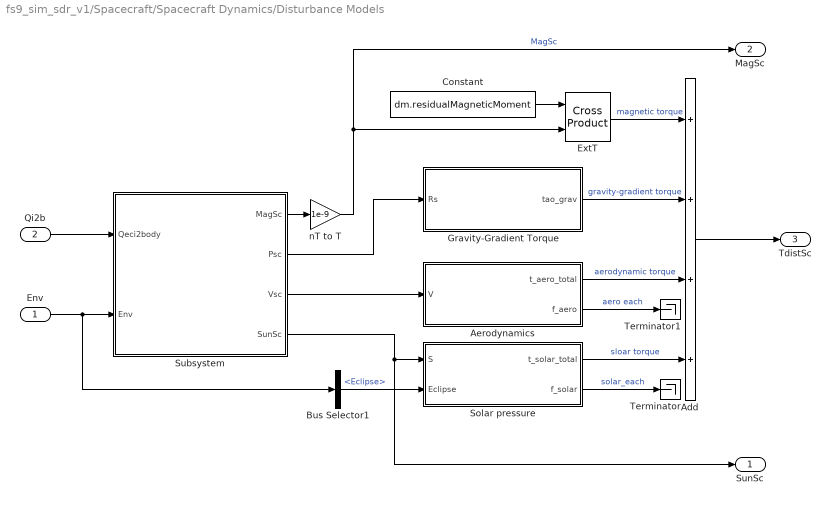
== system fs9_sim_sdr_v1/Spacecraft/Spacecraft Dynamics/Disturbance Models ==
  Env : Inport
  Qi2b : Inport  Port=2
  Add : Sum  Inputs=4
  Aerodynamics : MATLAB Function  TreatAsAtomicUnit=on
  Bus Selector1 : BusSelector  OutputSignals=Eclipse
  Constant : Constant  Value=dm.residualMagneticMoment
  ExtT : vrlib/Utilities/Cross Product
  Gravity-Gradient Torque : MATLAB Function  TreatAsAtomicUnit=on
  Solar pressure : MATLAB Function  TreatAsAtomicUnit=on
  Subsystem : Subsystem
  Terminator : Terminator
  Terminator1 : Terminator
  nT to T : Gain  Gain=1e-9
  SunSc : Outport
  MagSc : Outport  Port=2
  TdistSc : Outport  Port=3
  wires:
  Gravity-Gradient Torque/1(tao_grav) -> Add/2  "gravity-gradient torque"
  Add/1 -> TdistSc/1
  Aerodynamics/2(f_aero) -> Terminator1/1  "aero each"
  Solar pressure/2(f_solar) -> Terminator/1  "solar_each"
  Env/1 -> Subsystem/2(Env), Bus Selector1/1
  Bus Selector1/1 -> Solar pressure/2(Eclipse)  "<Eclipse>"
  Qi2b/1 -> Subsystem/1(Qeci2body)
  Subsystem/2(Psc) -> Gravity-Gradient Torque/1(Rs)
  Subsystem/3(Vsc) -> Aerodynamics/1(V)
  Subsystem/4(SunSc) -> SunSc/1, Solar pressure/1(S)
  Aerodynamics/1(t_aero_total) -> Add/3  "aerodynamic torque"
  Solar pressure/1(t_solar_total) -> Add/4  "sloar torque"
  Constant/1 -> ExtT/1
  Subsystem/1(MagSc) -> nT to T/1
  ExtT/1 -> Add/1  "magnetic torque"
  nT to T/1 -> MagSc/1, ExtT/2  "MagSc"

== system fs9_sim_sdr_v1/Spacecraft/Spacecraft Dynamics/RigidBody Dynamics ==
  N : Inport
  h : Inport  Port=2
  Constant : Constant  Value=dm.L0
  Constant3 : Constant  Value=dm.Qi2b0
  Integrator : Integrator  InitialConditionSource=external
  Integrator1 : Integrator  InitialConditionSource=external
  MATLAB Function1 : MATLAB Function  TreatAsAtomicUnit=on
  MATLAB Function2 : MATLAB Function  TreatAsAtomicUnit=on
  MATLAB Function3 : MATLAB Function  TreatAsAtomicUnit=on
  QNoramlize : Subsystem
  To Workspace : ToWorkspace  VariableName=TrueQuatEci2Body  SaveFormat=Timeseries  SampleTime=-1
  Qi2b : Outport  VectorParamsAs1DForOutWhenUnconnected=off
  Wb : Outport  Port=2  VectorParamsAs1DForOutWhenUnconnected=off
  wires:
  Constant/1 -> Integrator/2
  N/1 -> MATLAB Function1/2(N)
  MATLAB Function1/1(dLdt) -> Integrator/1
  MATLAB Function3/1(dQdt) -> Integrator1/1
  Constant3/1 -> Integrator1/2
  MATLAB Function2/1(W) -> MATLAB Function3/2(W), Wb/1, MATLAB Function1/3(W)
  Integrator/1 -> MATLAB Function2/2(L)  "Lb"
  h/1 -> MATLAB Function2/1(h), MATLAB Function1/1(h)
  Integrator1/1 -> QNoramlize/1(Qin)
  QNoramlize/1(Qunit) -> Qi2b/1, To Workspace/1, MATLAB Function3/1(Qi2b)

== system fs9_sim_sdr_v1/Space Environment Models/MagneticField/Variant Subsystem/IGRF2020 ==
  Pecf : Inport
  Constant : Constant  Commented=on  Value=dm.epoch.utc(1)
  Demux : Demux  Outputs=2
  Direction Cosine Matrix ECEF to NED : aerolibtransform2/Direction Cosine Matrix ECEF to NED
  ECEF Position to LLA : ECEF2LLA  R=6378137
  IGRF_ned2ecef : MATLAB Function  TreatAsAtomicUnit=on
  International Geomagnetic Reference Field : IGRF  time_in=off  month=June  day=21  year=2023
      settings: AttributesFormatString=%<generation>
  Mux1 : Mux  Inputs=9
  Scope : Scope
  Terminator : Terminator
  To Workspace : ToWorkspace  Commented=on  VariableName=MagEcef7Days  SaveFormat=Timeseries  SampleTime=-1
  BnT : Outport  VectorParamsAs1DForOutWhenUnconnected=off
  wires:
  International Geomagnetic Reference Field/7 -> Mux1/6
  International Geomagnetic Reference Field/4 -> Mux1/3
  International Geomagnetic Reference Field/3 -> Mux1/2
  International Geomagnetic Reference Field/6 -> Mux1/5
  International Geomagnetic Reference Field/5 -> Mux1/4
  International Geomagnetic Reference Field/9 -> Mux1/8
  International Geomagnetic Reference Field/8 -> Mux1/7
  International Geomagnetic Reference Field/10 -> Mux1/9
  Pecf/1 -> ECEF Position to LLA/1
  Mux1/1 -> Terminator/1
  International Geomagnetic Reference Field/2 -> Mux1/1
  ECEF Position to LLA/1 -> Demux/1, Direction Cosine Matrix ECEF to NED/1
  ECEF Position to LLA/2 -> International Geomagnetic Reference Field/1
  Demux/1 -> International Geomagnetic Reference Field/2
  Demux/2 -> International Geomagnetic Reference Field/3
  Direction Cosine Matrix ECEF to NED/1 -> IGRF_ned2ecef/1(DCM)
  IGRF_ned2ecef/1(Vecef) -> To Workspace/1, BnT/1
  International Geomagnetic Reference Field/1 -> IGRF_ned2ecef/2(Vned), Scope/1

== system fs9_sim_sdr_v1/Space Environment Models/Orbit Propagator /gravityField/J2 ==
  Integrator2 : Integrator  InitialConditionSource=external
  J2 Jack : MATLAB Function  TreatAsAtomicUnit=on
  PV2 : Constant  Value=dm.init_pv_eci
  PV : Outport
  wires:
  Integrator2/1 -> PV/1, J2 Jack/1(X)  "J2"
  J2 Jack/1(Xdot) -> Integrator2/1
  PV2/1 -> Integrator2/2

== system fs9_sim_sdr_v1/Space Environment Models/Orbit Propagator /gravityField/TwoBodyRHS ==
  Integrator : Integrator  InitialConditionSource=external
  MATLAB Function : MATLAB Function  TreatAsAtomicUnit=on
  PV0 : Constant  Value=dm.init_pv_eci
  PV : Outport
  wires:
  Integrator/1 -> PV/1, MATLAB Function/1(X)  "TwoBody"
  MATLAB Function/1(Xdot) -> Integrator/1
  PV0/1 -> Integrator/2

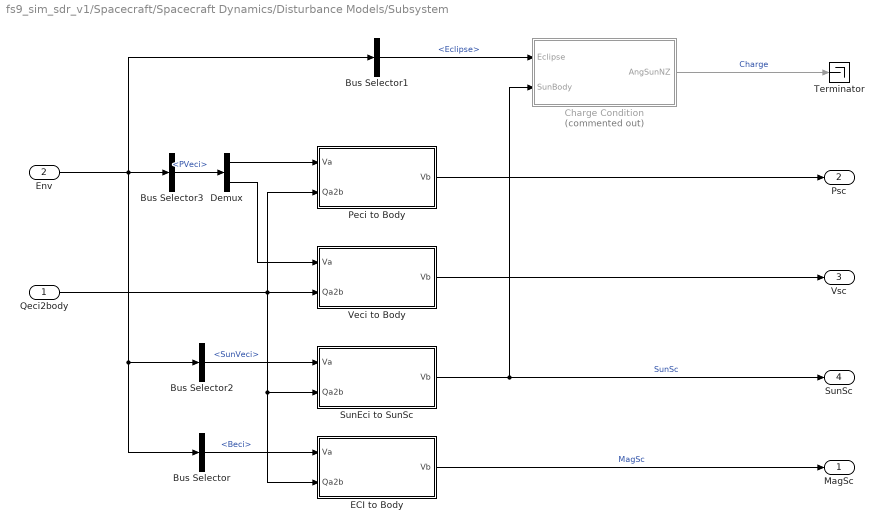
== system fs9_sim_sdr_v1/Spacecraft/Spacecraft Dynamics/Disturbance Models/Subsystem ==
  Qeci2body : Inport
  Env : Inport  Port=2
  Bus Selector : BusSelector  OutputSignals=Beci
  Bus Selector1 : BusSelector  OutputSignals=Eclipse
  Bus Selector2 : BusSelector  OutputSignals=SunVeci
  Bus Selector3 : BusSelector  OutputSignals=PVeci
  Charge Condition : MATLAB Function  Commented=on  TreatAsAtomicUnit=on
  Demux : Demux  Outputs=2
  ECI to Body : MATLAB Function  TreatAsAtomicUnit=on
  Peci to Body : MATLAB Function  TreatAsAtomicUnit=on
  SunEci to SunSc : MATLAB Function  TreatAsAtomicUnit=on
  Terminator : Terminator
  Veci to Body : MATLAB Function  TreatAsAtomicUnit=on
  MagSc : Outport
  Psc : Outport  Port=2
  Vsc : Outport  Port=3
  SunSc : Outport  Port=4
  wires:
  Qeci2body/1 -> ECI to Body/2(Qa2b), SunEci to SunSc/2(Qa2b), Peci to Body/2(Qa2b), Veci to Body/2(Qa2b)
  Bus Selector/1 -> ECI to Body/1(Va)  "<Beci>"
  Peci to Body/1(Vb) -> Psc/1
  Bus Selector2/1 -> SunEci to SunSc/1(Va)  "<SunVeci>"
  ECI to Body/1(Vb) -> MagSc/1  "MagSc"
  Env/1 -> Bus Selector1/1, Bus Selector3/1, Bus Selector/1, Bus Selector2/1
  SunEci to SunSc/1(Vb) -> Charge Condition/2(SunBody), SunSc/1  "SunSc"
  Veci to Body/1(Vb) -> Vsc/1
  Bus Selector3/1 -> Demux/1  "<PVeci>"
  Demux/1 -> Peci to Body/1(Va)
  Demux/2 -> Veci to Body/1(Va)
  Bus Selector1/1 -> Charge Condition/1(Eclipse)  "<Eclipse>"
  Charge Condition/1(AngSunNZ) -> Terminator/1  "Charge"

== system fs9_sim_sdr_v1/Spacecraft/Spacecraft Dynamics/RigidBody Dynamics/QNoramlize ==
  Qin : Inport
  Assertion : Assertion
  Divide : Product  Inputs=*/
  VectorNorm : Subsystem
  Qunit : Outport
  wires:
  Qin/1 -> VectorNorm/1(V), Divide/1
  Divide/1 -> Qunit/1
  VectorNorm/1(normV) -> Assertion/1, Divide/2

== system fs9_sim_sdr_v1/Spacecraft/Spacecraft Dynamics/RigidBody Dynamics/QNoramlize/VectorNorm ==
  V : Inport
  Dot Product1 : DotProduct  OutDataTypeStr=Inherit: Inherit via internal rule
  Square Root1 : Sqrt
  normV : Outport
  wires:
  Dot Product1/1 -> Square Root1/1
  V/1 -> Dot Product1/2, Dot Product1/1
  Square Root1/1 -> normV/1

== matlab function fs9_sim_sdr_v1/Space Environment Models/ECI2ECF ==
  data: Rf2i output; jdut1 input; Pecf output; Peci input
%% ECI to ECEF Transformation
function [Rf2i, Pecf]  = ECI2ECF(jdut1, Peci)
Ri2f  = R3(JD2GMST(jdut1));
Pecf  = Ri2f*Peci; %in m
Rf2i  = Ri2f';

== matlab function fs9_sim_sdr_v1/Space Environment Models/Orbit Propagator /MATLAB Function ==
  data: X input; Xdot output; dm parameter
function Xdot = TwoBodyRHS(X, dm)

r = X(1:3);
v = X(4:6);
Xdot=[v; -(dm.mu_e*r/norm(r)^3)];

== matlab function fs9_sim_sdr_v1/Space Environment Models/MagneticField/Variant Subsystem/MagneticDipoleModel ==
  data: Pecf input; BnT output; dm parameter
function BnT = MagDipole(Pecf, dm)

BnT = MagneticDipole(Pecf, dm.mpm);

== matlab function fs9_sim_sdr_v1/Spacecraft/Spacecraft Dynamics/Disturbance Models/Aerodynamics ==
  data: t_aero_total output; f_aero output; V input; dm parameter
function [t_aero_total, f_aero] = Aerodynamics(V,dm)
    f_aero = zeros(length(dm.norV),3);
    t_aero = zeros(length(dm.norV),3);
    for i = 1:length(dm.norV)
        if dot(dm.norV(i,:),V)>0
        f_aero(i,:) = -0.5 * dm.aeroCoeffDrag * dm.airDensity * norm(V)^2 * dm.area(i)*1e-6 * dot(dm.norV(i,:),V/norm(V)) *V/norm(V);
        t_aero(i,:) = cross(dm.rs(i,:),f_aero(i,:));
        end    
    end
     t_aero_total = sum(t_aero)';
end

== matlab function fs9_sim_sdr_v1/Spacecraft/Spacecraft Dynamics/Disturbance Models/Gravity-Gradient Torque ==
  data: Rs input; tao_grav output; dm parameter
function tao_grav = dist_gravity(Rs, dm)

% from Wertx p567
% Rs_hat = ECI Position unit vector in body frame
Rs_hat = -Rs/norm(Rs);
tao_grav = ((3*dm.mu_e/norm(Rs)^3)*cross(Rs_hat, dm.Ib*Rs_hat));

== matlab function fs9_sim_sdr_v1/Spacecraft/Spacecraft Dynamics/Disturbance Models/Solar pressure ==
  data: t_solar_total output; f_solar output; S input; dm parameter; Eclipse input
function [t_solar_total,f_solar ] = SolarPressure(S,dm, Eclipse)
    f_solar = zeros(length(dm.norV),3);
    t_solar = zeros(length(dm.norV),3);
    if Eclipse ==0
        for i = 1:length(dm.norV)
            if dot(dm.norV(i,:),S)>0
            f_solar(i,:) = -dm.P*dm.area(i)*1e-6*dot(dm.norV(i,:),S)*...
                ((1-dm.Cs)*S' + 2*(dm.Cd/3 + dm.Cs*dot(dm.norV(i,:),S))*dm.norV(i,:));
            t_solar(i,:) = cross(dm.rs(i,:),f_solar(i,:));
            end
        end
    end
    t_solar_total = sum(t_solar)';
end

== matlab function fs9_sim_sdr_v1/Spacecraft/Spacecraft Dynamics/Disturbance Models/Subsystem/ECI to Body ==
  data: Va input; Qa2b input; Vb output
function Vb = EciToBody(Va,Qa2b)
Qb2a = QInv(Qa2b);
qout = QMul(QMul(Qb2a, [0;Va]), Qa2b);
Vb   = [qout(2) qout(3) qout(4)]';

== matlab function fs9_sim_sdr_v1/RW_CTRL_FUN/Angular momentum Estimate ==
  settings: updateMethod=DISCRETE
  data: w_rpm input; tc input; h output; fsw parameter
function h = fcn(w_rpm,tc, fsw) %[C0, h]
persistent hrw

if isempty(hrw)
    hrw = fsw.rw.eqpt.H0;
end

rpm2rads    = (2*pi)/60;
J           = fsw.rw.eqpt.MOI; %parm(1); % 0.00663; %kg-m2 from 2ICD2885 Rev C August 2019
Te          = fsw.dt; %parm(2); % control period
w_est       = 0.52/10;

w = w_rpm*rpm2rads; 
h = hrw + 1.4 * w_est *Te*(J.*w-hrw);
hrw = h + Te*tc;
% h = J*w-h0;

== matlab function fs9_sim_sdr_v1/Spacecraft/Spacecraft Dynamics/Disturbance Models/Subsystem/SunEci to SunSc ==
  data: Va input; Qa2b input; Vb output
function Vb = EciToBody(Va,Qa2b)
Qb2a = QInv(Qa2b);
qout = QMul(QMul(Qb2a, [0;Va]), Qa2b);
Vb   = [qout(2) qout(3) qout(4)]';

== matlab function fs9_sim_sdr_v1/RW_CTRL_FUN/ComputeSaturate ==
  data: T input; Tc output; fsw parameter
function Tc = TorqueSaturation(T, fsw)
T0   = fsw.DeltaTalloc;%fsw.rw.func.maxTorque;
Trw  = abs(T');
maxT = max(Trw);
if maxT > T0
    Tc = (T0/maxT).*T;
else
    Tc = T;
end

== matlab function fs9_sim_sdr_v1/Sensor Modeling/MATLAB Function ==
  data: noise_ang input; SunSc input; SS_TM output; EclipFlag input; dm parameter
function SS_TM  = SunSensor(noise_ang, SunSc, EclipFlag, dm)
coder.extrinsic('randn');%%https://www.mathworks.com/matlabcentral/answers/385475-why-do-calls-to-randn-in-separate-matlab-function-blocks-return-the-same-sequence-of-random-number
if EclipFlag~=1
    %% Sun Sensor Modeling by Rotation
    %0.3 deg in 3-sigma from Solar MEMS type xx
     a1 = noise_ang(1);
     a2 = noise_ang(2);
     ca1 = cos(a1); sa1 = sin(a1);
     ca2 = cos(a2); sa2 = sin(a2);
     Rxy = [ca2       0        sa2;...
            sa1*sa2  ca1  -ca2*sa1;...
           -ca1*sa2  sa1   ca1*ca2];

    SunSc_noise = Rxy*SunSc;
    ang_ss1 = acos(dot(SunSc_noise, dm.ss1_mdl.los));
    ang_ss2 = acos(dot(SunSc_noise, dm.ss2_mdl.los));
    
    if ang_ss1 < dm.ss_mdl.fov || ang_ss2 < dm.ss_mdl.fov
        Valid = 1;
    else
        Valid = 0;
    end
else
    Valid = 0;
    SunSc_noise = zeros(3, 1);
end

SS_TM =[SunSc_noise; Valid];

end

% %% Eigen Axis Rotation by Rodrigues Rotation Formula
% function R = EigRotMatrix(n, theta)
% nx = [	0       -n(3)	n(2);...
%     n(3)	0       -n(1);...
%     -n(2)	n(1)    0	];
% R  = cos(theta)*eye(3)+(1-cos(theta))*(n*n')-sin(theta)*nx;
% end
